simulink model "AUV_Model"  (R2019b)
settings: Solver=VariableStepAuto  StartTime=0.0  StopTime=300  FixedStep=0.5  RelTol=1e-3
InitFcn:
  | mdlWks = get_param(gcs,'ModelWorkspace');
  | a = getVariable(mdlWks,'a');
  | b = getVariable(mdlWks,'b');
  | c = getVariable(mdlWks,'c');
StopFcn:
  | figure(2)
  | plot3(Position_Data(1,1),Position_Data(1,2),Position_Data(1,3),'r*')
  | hold on
  | plot3(Position_Data(:,1),Position_Data(:,2),Position_Data(:,3));
  | plot3(Position_Data(end,1),Position_Data(end,2),Position_Data(end,3),'g*');
  | grid on
  | legend('Start Point','Trajectory','End Point')
model workspace (MAT data in the model file):
  a = 1
  b = 0
  c = 1
undefined symbols (not defined in the file): sigbuilder_block
libraries: simulink x6, sharedtransform x6, vrlib x6, dspfdesign x6, shared6dof x1, aerolibasang x1, aerolibnav x1
(part 2 of 3)

== system AUV_Model/ Translation Controller ==
  Actual Parameters : Inport
  Reference Parameters : Inport  Port=2
  Position Controller : Subsystem  VariantControl=a==0
  Velocity Controller : Subsystem  VariantControl=a==1
  Thrust Control : Outport  VectorParamsAs1DForOutWhenUnconnected=off

== system AUV_Model/Plant and Environment Model ==
  Thrust Control : Inport
  Combine Forces and Moments : Subsystem
  Dynamics solver : Subsystem
  Environmental Forces & Moments : Subsystem
  Propulsion Forces & Moments : Subsystem
  Outport : Outport  VectorParamsAs1DForOutWhenUnconnected=off
  wires:
  Thrust Control/1 -> Propulsion Forces & Moments/1(Thrust Control In)
  Propulsion Forces & Moments/1(Propulsion Parameters) -> Combine Forces and Moments/1(Propulsion Parameters)
  Environmental Forces & Moments/1(Environment Parameters) -> Combine Forces and Moments/2(Hydrodynamic Force)
  Combine Forces and Moments/1(Total Force) -> Dynamics solver/1(Total Force)
  Combine Forces and Moments/2(Total Moment) -> Dynamics solver/2(Total Moment)
  Dynamics solver/1(AUV Data) -> Outport/1
  Dynamics solver/2(Internal Parameters) -> Environmental Forces & Moments/1(AOA_SideSlip)

== system AUV_Model/Sensor data and State Estimation ==
  AUV_Parameters : Inport
  System With Noise : Subsystem  VariantControl=b==0
  System without Noise : Subsystem  VariantControl=b==1
  Filtered Parameters : Outport  VectorParamsAs1DForOutWhenUnconnected=off

== system AUV_Model/Switch Parameters ==
  Constant : Constant  Value=a
  Constant1 : Constant  Value=b
  Constant2 : Constant  Value=c
  Terminator1 : Terminator
  Terminator2 : Terminator
  Terminator3 : Terminator
  wires:
  Constant/1 -> Terminator1/1
  Constant1/1 -> Terminator2/1
  Constant2/1 -> Terminator3/1

== system AUV_Model/Translational Reference ==
  Bus Creator : BusCreator  Inputs=2
  Constant : Constant  Value=-10
  Constant1 : Constant  Value=0
  Mux : Mux  Inputs=3
  Mux1 : Mux  Inputs=3
  Signal Builder : Subsystem  Tag=STV Subsys  LoadFcn=sigbuilder_block('load');  StartFcn=sigbuilder_block('start');  StopFcn=sigbuilder_block('stop');  ClipboardFcn=sigbuilder_block('clipboard');  mask(Sigbuilder block){tuvar=[0:10]}
      mask help: Simulink:masks:SigbuilderBlock_MD
      mask init:
      | if ~strcmp(get_param(bdroot(gcbh),'SimulationStatus'),'stopped') tuvar = sigbuilder_block('maskInit'); end
      settings: CopyFcn=sigbuilder_block('copy');  DeleteFcn=sigbuilder_block('delete');  ModelCloseFcn=sigbuilder_block('modelClose');  PreSaveFcn=sigbuilder_block('preSave');  PauseFcn=sigbuilder_block('pause');  ContinueFcn=sigbuilder_block('continue');  NameChangeFcn=sigbuilder_block('namechange');  OpenFcn=sigbuilder_block('open',[49.5 -20.25 1204.5 394.5 ]);  CloseFcn=sigbuilder_block('close');
      mask Display: plot(0, 0, 100, 100,[2, 2, 32, 32, 2], [68, 8, 8, 68, 68],[32, 2], [38, 38], [32, 19, 2],[53, 60, 44], [32, 17, 17, 2],[16, 16, 31, 31]);txt = getActiveGroup(gcbh);text(2, 100, txt,'verticalAlignment', 'top');
  Step : Step  Time=30  Before=0.2  After=0  SampleTime=0
  Step1 : Step  Time=150  After=5  SampleTime=0
  Reference Parameters : Outport  VectorParamsAs1DForOutWhenUnconnected=off
  wires:
  Mux/1 -> Bus Creator/1  "Reference Position"
  Constant/1 -> Mux/1, Mux/2
  Step1/1 -> Mux/3
  Mux1/1 -> Bus Creator/2  "Reference Velocity"
  Bus Creator/1 -> Reference Parameters/1
  Signal Builder/1(Signal 2) -> Mux1/3
  Constant1/1 -> Mux1/2
  Step/1 -> Mux1/1

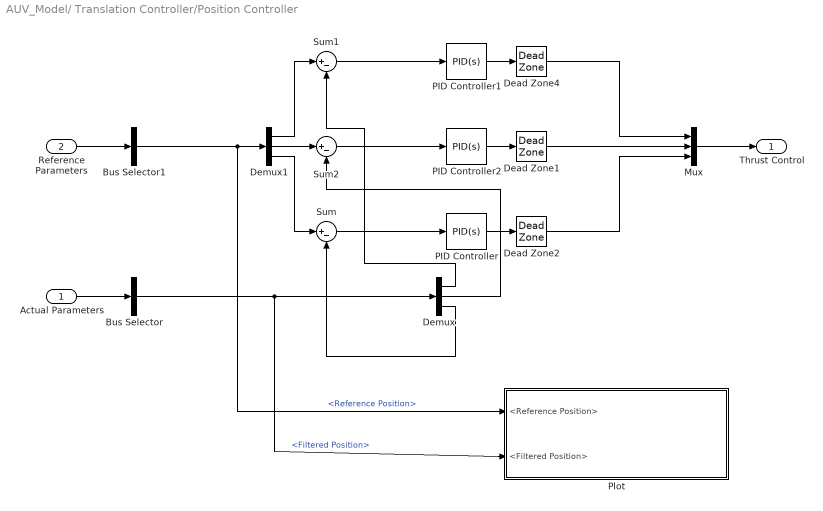
== system AUV_Model/ Translation Controller/Position Controller ==
  Actual Parameters : Inport
  Reference Parameters : Inport  Port=2
  Bus Selector : BusSelector  OutputSignals=Filtered Position
  Bus Selector1 : BusSelector  OutputSignals=Reference Position
  Dead Zone1 : DeadZone  LowerValue=-0.05  UpperValue=+0.05  SaturateOnIntegerOverflow=on
  Dead Zone2 : DeadZone  LowerValue=-0.05  UpperValue=+0.05  SaturateOnIntegerOverflow=on
  Dead Zone4 : DeadZone  LowerValue=-0.05  UpperValue=+0.05  SaturateOnIntegerOverflow=on
  Demux : Demux  Outputs=3
  Demux1 : Demux  Outputs=3
  Mux : Mux  Inputs=3
  PID Controller : simulink/Continuous/PID Controller  Controller=PID  Form=Parallel  TimeDomain=Continuous-time  SampleTime=-1  IntegratorMethod=Forward Euler  FilterMethod=Forward Euler  ControllerParametersSource=internal  P=-0.0440831016133051  I=-0.00046335965727533  D=-0.931852208113014  UseFilter=on  N=205.904485551143  TunerSelectOption=Transfer Function Based (PID Tuner App)  InitialConditionSource=internal  InitialConditionForIntegrator=0  InitialConditionForFilter=0  DifferentiatorICPrevScaledInput=0  ExternalReset=none  TrackingMode=off  Kt=1  LimitOutput=off  UpperSaturationLimit=inf  LowerSaturationLimit=-inf  LinearizeAsGain=on  AntiWindupMode=none  Kb=1  POutMin=[]  POutMax=[]  IOutMin=[]  IOutMax=[]  DOutMin=[]  DOutMax=[]  NOutMin=[]  NOutMax=[]  SumOutMin=[]  SumOutMax=[]  SaturationOutMin=[]  SaturationOutMax=[]  PParamMin=[]  PParamMax=[]  IParamMin=[]  IParamMax=[]  DParamMin=[]  DParamMax=[]  NParamMin=[]  NParamMax=[]  KbParamMin=[]  KbParamMax=[]  KtParamMin=[]  KtParamMax=[]  KbOutMin=[]  KbOutMax=[]  KtOutMin=[]  KtOutMax=[]  IntegratorOutMin=[]  IntegratorOutMax=[]  FilterOutMin=[]  FilterOutMax=[]  SumI1OutMin=[]  SumI1OutMax=[]  SumI2OutMin=[]  SumI2OutMax=[]  SumI3OutMin=[]  SumI3OutMax=[]  SumI4OutMin=[]  SumI4OutMax=[]  SumDOutMin=[]  SumDOutMax=[]  DifferentiatorOutMin=[]  DifferentiatorOutMax=[]  FilterDiffOutCoefMin=[]  FilterDiffOutCoefMax=[]  ReciprocalOutMin=[]  ReciprocalOutMax=[]  SumDenOutMin=[]  SumDenOutMax=[]  SumNumOutMin=[]  SumNumOutMax=[]  DivideOutMin=[]  DivideOutMax=[]  IntegratorContinuousStateAttributes=''  IntegratorStateMustResolveToSignalObject=off  IntegratorRTWStateStorageClass=Auto  FilterContinuousStateAttributes=''  FilterStateMustResolveToSignalObject=off  FilterRTWStateStorageClass=Auto  ParallelPVariant=InternalParameters  IdealPVariant=Disabled  IVariant=InternalParameters  DVariant=InternalParameters  IntegratorVariant=Continuous  SatVariant=Disabled  AWVariant=Passthrough  PCopyVariant=Disabled  TRVariant=Disabled  FdbkBlocksVariant=Forward  IdealPFdbkVariant=Disabled  SatFdbkVariant=Disabled  DerivativeFilterVariant=ContFilter  NVariant=InternalParameters  NCopyVariant=Disabled  FilterICVariant=InternalICsFilter  IntegratorICVariant=InternalICs  ExternalResetVariant=Disabled  TRSumVariant=Passthrough  SumFdbkVariant=Disabled  SumVariant=Sum_PID
  PID Controller1 : simulink/Continuous/PID Controller  Controller=PID  Form=Parallel  TimeDomain=Continuous-time  SampleTime=-1  IntegratorMethod=Forward Euler  FilterMethod=Forward Euler  ControllerParametersSource=internal  P=0.0352909553215239  I=0.000468513300704798  D=0.59064410837381  UseFilter=on  N=260.062804539004  TunerSelectOption=Transfer Function Based (PID Tuner App)  InitialConditionSource=internal  InitialConditionForIntegrator=0  InitialConditionForFilter=0  DifferentiatorICPrevScaledInput=0  ExternalReset=none  TrackingMode=off  Kt=1  LimitOutput=off  UpperSaturationLimit=inf  LowerSaturationLimit=-inf  LinearizeAsGain=on  AntiWindupMode=none  Kb=1  POutMin=[]  POutMax=[]  IOutMin=[]  IOutMax=[]  DOutMin=[]  DOutMax=[]  NOutMin=[]  NOutMax=[]  SumOutMin=[]  SumOutMax=[]  SaturationOutMin=[]  SaturationOutMax=[]  PParamMin=[]  PParamMax=[]  IParamMin=[]  IParamMax=[]  DParamMin=[]  DParamMax=[]  NParamMin=[]  NParamMax=[]  KbParamMin=[]  KbParamMax=[]  KtParamMin=[]  KtParamMax=[]  KbOutMin=[]  KbOutMax=[]  KtOutMin=[]  KtOutMax=[]  IntegratorOutMin=[]  IntegratorOutMax=[]  FilterOutMin=[]  FilterOutMax=[]  SumI1OutMin=[]  SumI1OutMax=[]  SumI2OutMin=[]  SumI2OutMax=[]  SumI3OutMin=[]  SumI3OutMax=[]  SumI4OutMin=[]  SumI4OutMax=[]  SumDOutMin=[]  SumDOutMax=[]  DifferentiatorOutMin=[]  DifferentiatorOutMax=[]  FilterDiffOutCoefMin=[]  FilterDiffOutCoefMax=[]  ReciprocalOutMin=[]  ReciprocalOutMax=[]  SumDenOutMin=[]  SumDenOutMax=[]  SumNumOutMin=[]  SumNumOutMax=[]  DivideOutMin=[]  DivideOutMax=[]  IntegratorContinuousStateAttributes=''  IntegratorStateMustResolveToSignalObject=off  IntegratorRTWStateStorageClass=Auto  FilterContinuousStateAttributes=''  FilterStateMustResolveToSignalObject=off  FilterRTWStateStorageClass=Auto  ParallelPVariant=InternalParameters  IdealPVariant=Disabled  IVariant=InternalParameters  DVariant=InternalParameters  IntegratorVariant=Continuous  SatVariant=Disabled  AWVariant=Passthrough  PCopyVariant=Disabled  TRVariant=Disabled  FdbkBlocksVariant=Forward  IdealPFdbkVariant=Disabled  SatFdbkVariant=Disabled  DerivativeFilterVariant=ContFilter  NVariant=InternalParameters  NCopyVariant=Disabled  FilterICVariant=InternalICsFilter  IntegratorICVariant=InternalICs  ExternalResetVariant=Disabled  TRSumVariant=Passthrough  SumFdbkVariant=Disabled  SumVariant=Sum_PID
  PID Controller2 : simulink/Continuous/PID Controller  Controller=PID  Form=Parallel  TimeDomain=Continuous-time  SampleTime=-1  IntegratorMethod=Forward Euler  FilterMethod=Forward Euler  ControllerParametersSource=internal  P=0.172975950646219  I=0.00387308418128247  D=1.71646711354372  UseFilter=on  N=438.622536688858  TunerSelectOption=Transfer Function Based (PID Tuner App)  InitialConditionSource=internal  InitialConditionForIntegrator=0  InitialConditionForFilter=0  DifferentiatorICPrevScaledInput=0  ExternalReset=none  TrackingMode=off  Kt=1  LimitOutput=off  UpperSaturationLimit=inf  LowerSaturationLimit=-inf  LinearizeAsGain=on  AntiWindupMode=none  Kb=1  POutMin=[]  POutMax=[]  IOutMin=[]  IOutMax=[]  DOutMin=[]  DOutMax=[]  NOutMin=[]  NOutMax=[]  SumOutMin=[]  SumOutMax=[]  SaturationOutMin=[]  SaturationOutMax=[]  PParamMin=[]  PParamMax=[]  IParamMin=[]  IParamMax=[]  DParamMin=[]  DParamMax=[]  NParamMin=[]  NParamMax=[]  KbParamMin=[]  KbParamMax=[]  KtParamMin=[]  KtParamMax=[]  KbOutMin=[]  KbOutMax=[]  KtOutMin=[]  KtOutMax=[]  IntegratorOutMin=[]  IntegratorOutMax=[]  FilterOutMin=[]  FilterOutMax=[]  SumI1OutMin=[]  SumI1OutMax=[]  SumI2OutMin=[]  SumI2OutMax=[]  SumI3OutMin=[]  SumI3OutMax=[]  SumI4OutMin=[]  SumI4OutMax=[]  SumDOutMin=[]  SumDOutMax=[]  DifferentiatorOutMin=[]  DifferentiatorOutMax=[]  FilterDiffOutCoefMin=[]  FilterDiffOutCoefMax=[]  ReciprocalOutMin=[]  ReciprocalOutMax=[]  SumDenOutMin=[]  SumDenOutMax=[]  SumNumOutMin=[]  SumNumOutMax=[]  DivideOutMin=[]  DivideOutMax=[]  IntegratorContinuousStateAttributes=''  IntegratorStateMustResolveToSignalObject=off  IntegratorRTWStateStorageClass=Auto  FilterContinuousStateAttributes=''  FilterStateMustResolveToSignalObject=off  FilterRTWStateStorageClass=Auto  ParallelPVariant=InternalParameters  IdealPVariant=Disabled  IVariant=InternalParameters  DVariant=InternalParameters  IntegratorVariant=Continuous  SatVariant=Disabled  AWVariant=Passthrough  PCopyVariant=Disabled  TRVariant=Disabled  FdbkBlocksVariant=Forward  IdealPFdbkVariant=Disabled  SatFdbkVariant=Disabled  DerivativeFilterVariant=ContFilter  NVariant=InternalParameters  NCopyVariant=Disabled  FilterICVariant=InternalICsFilter  IntegratorICVariant=InternalICs  ExternalResetVariant=Disabled  TRSumVariant=Passthrough  SumFdbkVariant=Disabled  SumVariant=Sum_PID
  Plot : Subsystem
  Sum : Sum  Inputs=|+-
  Sum1 : Sum  Inputs=|+-
  Sum2 : Sum  Inputs=|+-
  Thrust Control : Outport  VectorParamsAs1DForOutWhenUnconnected=off
  wires:
  Demux1/1 -> Sum1/1
  Demux1/3 -> Sum/1
  Demux1/2 -> Sum2/1
  PID Controller1/1 -> Dead Zone4/1
  Demux/3 -> Sum/2
  PID Controller2/1 -> Dead Zone1/1
  Demux/2 -> Sum2/2
  Sum2/1 -> PID Controller2/1
  Demux/1 -> Sum1/2
  Sum/1 -> PID Controller/1
  PID Controller/1 -> Dead Zone2/1
  Sum1/1 -> PID Controller1/1
  Mux/1 -> Thrust Control/1
  Dead Zone4/1 -> Mux/1
  Dead Zone1/1 -> Mux/2
  Dead Zone2/1 -> Mux/3
  Actual Parameters/1 -> Bus Selector/1
  Bus Selector/1 -> Plot/2(<Filtered Position>), Demux/1  "<Filtered Position>"
  Reference Parameters/1 -> Bus Selector1/1
  Bus Selector1/1 -> Plot/1(<Reference Position>), Demux1/1  "<Reference Position>"

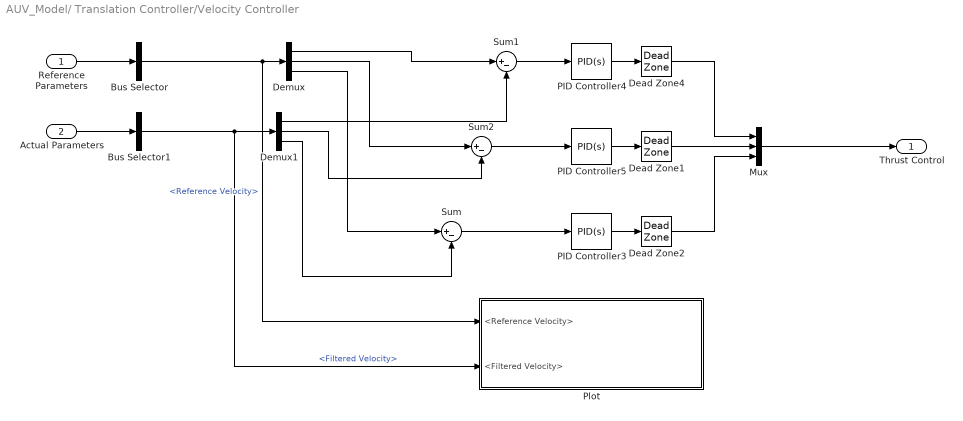
== system AUV_Model/ Translation Controller/Velocity Controller ==
  Reference Parameters : Inport
  Actual Parameters : Inport  Port=2
  Bus Selector : BusSelector  OutputSignals=Reference Velocity
  Bus Selector1 : BusSelector  OutputSignals=Filtered Velocity
  Dead Zone1 : DeadZone  LowerValue=-0.05  UpperValue=+0.05  SaturateOnIntegerOverflow=on
  Dead Zone2 : DeadZone  LowerValue=-0.05  UpperValue=+0.05  SaturateOnIntegerOverflow=on
  Dead Zone4 : DeadZone  LowerValue=-0.05  UpperValue=+0.05  SaturateOnIntegerOverflow=on
  Demux : Demux  Outputs=3
  Demux1 : Demux  Outputs=3
  Mux : Mux  Inputs=3
  PID Controller3 : simulink/Continuous/PID Controller  Controller=PID  Form=Parallel  TimeDomain=Continuous-time  SampleTime=-1  IntegratorMethod=Forward Euler  FilterMethod=Forward Euler  ControllerParametersSource=internal  P=-0.61964554396314  I=-0.140214385843897  D=0.00440045709674139  UseFilter=on  N=140.813904178727  TunerSelectOption=Transfer Function Based (PID Tuner App)  InitialConditionSource=internal  InitialConditionForIntegrator=0  InitialConditionForFilter=0  DifferentiatorICPrevScaledInput=0  ExternalReset=none  TrackingMode=off  Kt=1  LimitOutput=off  UpperSaturationLimit=inf  LowerSaturationLimit=-inf  LinearizeAsGain=on  AntiWindupMode=none  Kb=1  POutMin=[]  POutMax=[]  IOutMin=[]  IOutMax=[]  DOutMin=[]  DOutMax=[]  NOutMin=[]  NOutMax=[]  SumOutMin=[]  SumOutMax=[]  SaturationOutMin=[]  SaturationOutMax=[]  PParamMin=[]  PParamMax=[]  IParamMin=[]  IParamMax=[]  DParamMin=[]  DParamMax=[]  NParamMin=[]  NParamMax=[]  KbParamMin=[]  KbParamMax=[]  KtParamMin=[]  KtParamMax=[]  KbOutMin=[]  KbOutMax=[]  KtOutMin=[]  KtOutMax=[]  IntegratorOutMin=[]  IntegratorOutMax=[]  FilterOutMin=[]  FilterOutMax=[]  SumI1OutMin=[]  SumI1OutMax=[]  SumI2OutMin=[]  SumI2OutMax=[]  SumI3OutMin=[]  SumI3OutMax=[]  SumI4OutMin=[]  SumI4OutMax=[]  SumDOutMin=[]  SumDOutMax=[]  DifferentiatorOutMin=[]  DifferentiatorOutMax=[]  FilterDiffOutCoefMin=[]  FilterDiffOutCoefMax=[]  ReciprocalOutMin=[]  ReciprocalOutMax=[]  SumDenOutMin=[]  SumDenOutMax=[]  SumNumOutMin=[]  SumNumOutMax=[]  DivideOutMin=[]  DivideOutMax=[]  IntegratorContinuousStateAttributes=''  IntegratorStateMustResolveToSignalObject=off  IntegratorRTWStateStorageClass=Auto  FilterContinuousStateAttributes=''  FilterStateMustResolveToSignalObject=off  FilterRTWStateStorageClass=Auto  ParallelPVariant=InternalParameters  IdealPVariant=Disabled  IVariant=InternalParameters  DVariant=InternalParameters  IntegratorVariant=Continuous  SatVariant=Disabled  AWVariant=Passthrough  PCopyVariant=Disabled  TRVariant=Disabled  FdbkBlocksVariant=Forward  IdealPFdbkVariant=Disabled  SatFdbkVariant=Disabled  DerivativeFilterVariant=ContFilter  NVariant=InternalParameters  NCopyVariant=Disabled  FilterICVariant=InternalICsFilter  IntegratorICVariant=InternalICs  ExternalResetVariant=Disabled  TRSumVariant=Passthrough  SumFdbkVariant=Disabled  SumVariant=Sum_PID
  PID Controller4 : simulink/Continuous/PID Controller  Controller=PID  Form=Parallel  TimeDomain=Continuous-time  SampleTime=-1  IntegratorMethod=Forward Euler  FilterMethod=Forward Euler  ControllerParametersSource=internal  P=0.262050505979025  I=0.0518732197045156  D=-0.0235509594288088  UseFilter=on  N=11.1269567072699  TunerSelectOption=Transfer Function Based (PID Tuner App)  InitialConditionSource=internal  InitialConditionForIntegrator=0  InitialConditionForFilter=0  DifferentiatorICPrevScaledInput=0  ExternalReset=none  TrackingMode=off  Kt=1  LimitOutput=off  UpperSaturationLimit=inf  LowerSaturationLimit=-inf  LinearizeAsGain=on  AntiWindupMode=none  Kb=1  POutMin=[]  POutMax=[]  IOutMin=[]  IOutMax=[]  DOutMin=[]  DOutMax=[]  NOutMin=[]  NOutMax=[]  SumOutMin=[]  SumOutMax=[]  SaturationOutMin=[]  SaturationOutMax=[]  PParamMin=[]  PParamMax=[]  IParamMin=[]  IParamMax=[]  DParamMin=[]  DParamMax=[]  NParamMin=[]  NParamMax=[]  KbParamMin=[]  KbParamMax=[]  KtParamMin=[]  KtParamMax=[]  KbOutMin=[]  KbOutMax=[]  KtOutMin=[]  KtOutMax=[]  IntegratorOutMin=[]  IntegratorOutMax=[]  FilterOutMin=[]  FilterOutMax=[]  SumI1OutMin=[]  SumI1OutMax=[]  SumI2OutMin=[]  SumI2OutMax=[]  SumI3OutMin=[]  SumI3OutMax=[]  SumI4OutMin=[]  SumI4OutMax=[]  SumDOutMin=[]  SumDOutMax=[]  DifferentiatorOutMin=[]  DifferentiatorOutMax=[]  FilterDiffOutCoefMin=[]  FilterDiffOutCoefMax=[]  ReciprocalOutMin=[]  ReciprocalOutMax=[]  SumDenOutMin=[]  SumDenOutMax=[]  SumNumOutMin=[]  SumNumOutMax=[]  DivideOutMin=[]  DivideOutMax=[]  IntegratorContinuousStateAttributes=''  IntegratorStateMustResolveToSignalObject=off  IntegratorRTWStateStorageClass=Auto  FilterContinuousStateAttributes=''  FilterStateMustResolveToSignalObject=off  FilterRTWStateStorageClass=Auto  ParallelPVariant=InternalParameters  IdealPVariant=Disabled  IVariant=InternalParameters  DVariant=InternalParameters  IntegratorVariant=Continuous  SatVariant=Disabled  AWVariant=Passthrough  PCopyVariant=Disabled  TRVariant=Disabled  FdbkBlocksVariant=Forward  IdealPFdbkVariant=Disabled  SatFdbkVariant=Disabled  DerivativeFilterVariant=ContFilter  NVariant=InternalParameters  NCopyVariant=Disabled  FilterICVariant=InternalICsFilter  IntegratorICVariant=InternalICs  ExternalResetVariant=Disabled  TRSumVariant=Passthrough  SumFdbkVariant=Disabled  SumVariant=Sum_PID
  PID Controller5 : simulink/Continuous/PID Controller  Controller=PID  Form=Parallel  TimeDomain=Continuous-time  SampleTime=-1  IntegratorMethod=Forward Euler  FilterMethod=Forward Euler  ControllerParametersSource=internal  P=1.14371295451496  I=0.548529610159355  D=-0.00383210771245667  UseFilter=on  N=298.455325458939  TunerSelectOption=Transfer Function Based (PID Tuner App)  InitialConditionSource=internal  InitialConditionForIntegrator=0  InitialConditionForFilter=0  DifferentiatorICPrevScaledInput=0  ExternalReset=none  TrackingMode=off  Kt=1  LimitOutput=off  UpperSaturationLimit=inf  LowerSaturationLimit=-inf  LinearizeAsGain=on  AntiWindupMode=none  Kb=1  POutMin=[]  POutMax=[]  IOutMin=[]  IOutMax=[]  DOutMin=[]  DOutMax=[]  NOutMin=[]  NOutMax=[]  SumOutMin=[]  SumOutMax=[]  SaturationOutMin=[]  SaturationOutMax=[]  PParamMin=[]  PParamMax=[]  IParamMin=[]  IParamMax=[]  DParamMin=[]  DParamMax=[]  NParamMin=[]  NParamMax=[]  KbParamMin=[]  KbParamMax=[]  KtParamMin=[]  KtParamMax=[]  KbOutMin=[]  KbOutMax=[]  KtOutMin=[]  KtOutMax=[]  IntegratorOutMin=[]  IntegratorOutMax=[]  FilterOutMin=[]  FilterOutMax=[]  SumI1OutMin=[]  SumI1OutMax=[]  SumI2OutMin=[]  SumI2OutMax=[]  SumI3OutMin=[]  SumI3OutMax=[]  SumI4OutMin=[]  SumI4OutMax=[]  SumDOutMin=[]  SumDOutMax=[]  DifferentiatorOutMin=[]  DifferentiatorOutMax=[]  FilterDiffOutCoefMin=[]  FilterDiffOutCoefMax=[]  ReciprocalOutMin=[]  ReciprocalOutMax=[]  SumDenOutMin=[]  SumDenOutMax=[]  SumNumOutMin=[]  SumNumOutMax=[]  DivideOutMin=[]  DivideOutMax=[]  IntegratorContinuousStateAttributes=''  IntegratorStateMustResolveToSignalObject=off  IntegratorRTWStateStorageClass=Auto  FilterContinuousStateAttributes=''  FilterStateMustResolveToSignalObject=off  FilterRTWStateStorageClass=Auto  ParallelPVariant=InternalParameters  IdealPVariant=Disabled  IVariant=InternalParameters  DVariant=InternalParameters  IntegratorVariant=Continuous  SatVariant=Disabled  AWVariant=Passthrough  PCopyVariant=Disabled  TRVariant=Disabled  FdbkBlocksVariant=Forward  IdealPFdbkVariant=Disabled  SatFdbkVariant=Disabled  DerivativeFilterVariant=ContFilter  NVariant=InternalParameters  NCopyVariant=Disabled  FilterICVariant=InternalICsFilter  IntegratorICVariant=InternalICs  ExternalResetVariant=Disabled  TRSumVariant=Passthrough  SumFdbkVariant=Disabled  SumVariant=Sum_PID
  Plot : Subsystem
  Sum : Sum  Inputs=|+-
  Sum1 : Sum  Inputs=|+-
  Sum2 : Sum  Inputs=|+-
  Thrust Control : Outport  VectorParamsAs1DForOutWhenUnconnected=off
  wires:
  Demux1/3 -> Sum/2
  PID Controller3/1 -> Dead Zone2/1
  Demux/3 -> Sum/1
  PID Controller4/1 -> Dead Zone4/1
  PID Controller5/1 -> Dead Zone1/1
  Demux/2 -> Sum2/1
  Dead Zone2/1 -> Mux/3
  Dead Zone1/1 -> Mux/2
  Demux/1 -> Sum1/1
  Demux1/1 -> Sum1/2
  Demux1/2 -> Sum2/2
  Dead Zone4/1 -> Mux/1
  Mux/1 -> Thrust Control/1
  Sum1/1 -> PID Controller4/1
  Sum2/1 -> PID Controller5/1
  Sum/1 -> PID Controller3/1
  Bus Selector/1 -> Plot/1(<Reference Velocity>), Demux/1  "<Reference Velocity>"
  Reference Parameters/1 -> Bus Selector/1
  Bus Selector1/1 -> Plot/2(<Filtered Velocity>), Demux1/1  "<Filtered Velocity>"
  Actual Parameters/1 -> Bus Selector1/1

== system AUV_Model/Plant and Environment Model/Combine Forces and Moments ==
  Propulsion Parameters : Inport
  Hydrodynamic Force : Inport  Port=2
  Bus Selector : BusSelector  OutputSignals=PropForce,PropMoment
  Bus Selector1 : BusSelector  OutputSignals=LDForce,HSForce,HS Moment
  Saturation : Saturate  UpperLimit=600  LowerLimit=-600
  Saturation1 : Saturate  UpperLimit=600  LowerLimit=-600
  Sum : Sum  Inputs=+++
  Sum1 : Sum  Inputs=|++
  Total Force : Outport  VectorParamsAs1DForOutWhenUnconnected=off
  Total Moment : Outport  Port=2  VectorParamsAs1DForOutWhenUnconnected=off
  wires:
  Bus Selector1/3 -> Sum1/2  "<HS Moment>"
  Bus Selector/2 -> Sum1/1  "<PropMoment>"
  Sum/1 -> Saturation/1
  Sum1/1 -> Total Moment/1
  Saturation1/1 -> Sum/2
  Saturation/1 -> Total Force/1
  Propulsion Parameters/1 -> Bus Selector/1
  Hydrodynamic Force/1 -> Bus Selector1/1
  Bus Selector/1 -> Sum/1  "<PropForce>"
  Bus Selector1/1 -> Saturation1/1  "<LDForce>"
  Bus Selector1/2 -> Sum/3  "<HSForce>"

== system AUV_Model/Plant and Environment Model/Dynamics solver ==
  Total Force : Inport
  Total Moment : Inport  Port=2
  6DOF (Euler Angles) : shared6dof/6DOF (Euler Angles)  units=Metric (MKS)  mtype=Fixed  rep=Euler Angles  xme_0=[0.01 .01 .01]  Vm_0=[0.01 0.01 0.001]  eul_0=[0.001 0.001 0.001]  pm_0=[0.001 0.001 0.001]  mass_0=10  mass_e=0.5  mass_f=2.0  inertia=10*eye(3)  inertia_e=eye(3)  inertia_f=2*eye(3)  k_quat=1.0  vre_flag=on  abi_flag=on  aMode=0  xme_statename=''  Vm_statename=''  eul_statename=''  quat_statename=''  pm_statename=''  mass_statename=''
      settings: SourceProductBaseCode=AE
  Bus Creator : BusCreator  Inputs=4
  Bus Creator1 : BusCreator  Inputs=3
  Post-Processing : Subsystem
  Terminator : Terminator
  Terminator1 : Terminator
  AUV Data : Outport  VectorParamsAs1DForOutWhenUnconnected=off
  Internal Parameters : Outport  Port=2  VectorParamsAs1DForOutWhenUnconnected=off
  wires:
  6DOF (Euler Angles)/6 -> Post-Processing/4(Body angular rates)  "Body_rates"
  Post-Processing/3("AOA, Side slip") -> Bus Creator1/2  "AOA_SS"
  6DOF (Euler Angles)/8 -> Post-Processing/6(Body Acceleration)  "Body_acc"
  Post-Processing/2(" Position") -> Bus Creator/2  "Position"
  6DOF (Euler Angles)/7 -> Post-Processing/5(Body angular accelerations)  "Body_ang_acc"
  6DOF (Euler Angles)/2 -> Post-Processing/2(Position (Reference Frame))  "Pos_Ref"
  6DOF (Euler Angles)/3 -> Post-Processing/3(Orientation angles)  "Body_Angles"
  Post-Processing/1(Velocity) -> Bus Creator/1  "Velocity"
  6DOF (Euler Angles)/1 -> Post-Processing/1(Velocity (Reference Frame))  "Velocity_Ref"
  6DOF (Euler Angles)/5 -> Bus Creator1/3, Post-Processing/7(Body velocity)  "Velocity_body"
  Post-Processing/4(Orientation Angles) -> Bus Creator1/1, Bus Creator/3  "Orientation Angles"
  Post-Processing/5(IMU Data) -> Bus Creator/4  "IMU Data"
  Total Force/1 -> 6DOF (Euler Angles)/1
  Total Moment/1 -> 6DOF (Euler Angles)/2
  Bus Creator/1 -> AUV Data/1
  Bus Creator1/1 -> Internal Parameters/1
  6DOF (Euler Angles)/4 -> Terminator/1
  6DOF (Euler Angles)/9 -> Terminator1/1

== system AUV_Model/Plant and Environment Model/Environmental Forces & Moments ==
  AOA_SideSlip : Inport
  Bus Creator : BusCreator  Inputs=3
  Bus Selector : BusSelector  OutputSignals=Velocity_body,AOA_SS,Orientation Angles
  Hydrodynamic Forces : Subsystem  Variant=on
  Hydrostatic Forces : Subsystem
  Environment Parameters : Outport  VectorParamsAs1DForOutWhenUnconnected=off
  wires:
  Hydrodynamic Forces/1("Force due to Lift, Drag") -> Bus Creator/1  "LDForce"
  Hydrostatic Forces/1(Hydrostatic Force) -> Bus Creator/2  "HSForce"
  Hydrostatic Forces/2(Hydrostatic Moment) -> Bus Creator/3  "HS Moment"
  Bus Creator/1 -> Environment Parameters/1
  AOA_SideSlip/1 -> Bus Selector/1
  Bus Selector/1 -> Hydrodynamic Forces/1("Submarine Velocity (Body Axis) ")  "<Velocity_body>"
  Bus Selector/2 -> Hydrodynamic Forces/2("AOA, Side Slip")  "<AOA_SS>"
  Bus Selector/3 -> Hydrostatic Forces/1(In1)  "<Orientation Angles>"

== system AUV_Model/Plant and Environment Model/Propulsion Forces & Moments ==
  Thrust Control In : Inport
  Bus Creator : BusCreator  Inputs=2
  Force and moments due to Thrust : Subsystem
  Input commands to Thrust : Subsystem
  Propulsion Parameters : Outport  VectorParamsAs1DForOutWhenUnconnected=off
  wires:
  Input commands to Thrust/1(Thrust values) -> Force and moments due to Thrust/1(Thrust Inputs)
  Thrust Control In/1 -> Input commands to Thrust/1(Thrust Control Inputs)
  Force and moments due to Thrust/1(Propulsion Force) -> Bus Creator/1  "PropForce"
  Force and moments due to Thrust/2(Propulsion Moment) -> Bus Creator/2  "PropMoment"
  Bus Creator/1 -> Propulsion Parameters/1

== system AUV_Model/Sensor data and State Estimation/System With Noise ==
  AUV_Parameters : Inport
  " Sensor (IMU)" : Subsystem
  Internal filter : Subsystem
  Filtered Parameters : Outport  VectorParamsAs1DForOutWhenUnconnected=off
  wires:
  AUV_Parameters/1 -> " Sensor (IMU)"/1(IMU Inputs)
  Internal filter/1(Filtered Parameters) -> Filtered Parameters/1
  " Sensor (IMU)"/1(IMU Measurements) -> Internal filter/1(Accel)

== system AUV_Model/Sensor data and State Estimation/System without Noise ==
  AUV_Parameters : Inport
  Bus Creator : BusCreator  Inputs=2
  Bus Selector : BusSelector  OutputSignals=Position,Velocity
  Gain : Gain
  Gain1 : Gain
  Filtered Parameters : Outport  VectorParamsAs1DForOutWhenUnconnected=off
  wires:
  Bus Creator/1 -> Filtered Parameters/1
  Bus Selector/2 -> Gain1/1  "<Velocity>"
  Bus Selector/1 -> Gain/1  "<Position>"
  Gain1/1 -> Bus Creator/2  "Filtered Velocity"
  Gain/1 -> Bus Creator/1  "Filtered Position"
  AUV_Parameters/1 -> Bus Selector/1

== system AUV_Model/Translational Reference/Signal Builder ==
  Demux : Demux  Tag=STV Demux  Outputs=1
  FromWs : FromWorkspace  Tag=STV FromWs  VariableName=tuvar  SampleTime=0
      SigBuilderData=|
      | common.afterFinalStr = 'Extrapolate'
      | common.sampleTime = 0
      | dataSet.timeRange = [0 300]
      | dataSet.name = 'Group 1'
      | sbobj.Groups.Name = 'Group 1'
      | sbobj.Groups.Signals.Name = 'Signal 2'
      | sbobj.Groups.Signals.XData = [0 150 150 180 180 300]
      | sbobj.Groups.Signals.YData = [0 0 0.2 0.2 0 0]
      | sbobj.Groups.TimeRange = [0 300]
  Signal 2 : Outport  Tag=STV Outport  VectorParamsAs1DForOutWhenUnconnected=off
  wires:
  FromWs/1 -> Demux/1
  Demux/1 -> Signal 2/1

== system AUV_Model/ Translation Controller/Position Controller/Plot ==
  <Reference Position> : Inport
  <Filtered Position> : Inport  Port=2
  Demux2 : Demux  Outputs=3
  Demux3 : Demux  Outputs=3
  Mux1 : Mux  Inputs=2
  Mux2 : Mux  Inputs=2
  Mux3 : Mux  Inputs=2
  Scope : Scope  NumInputPorts=3
  wires:
  Mux3/1 -> Scope/3
  Demux3/1 -> Mux1/2
  Demux3/2 -> Mux2/2
  Demux2/3 -> Mux3/1
  Mux2/1 -> Scope/2
  Mux1/1 -> Scope/1
  Demux2/2 -> Mux2/1
  Demux2/1 -> Mux1/1
  Demux3/3 -> Mux3/2
  <Reference Position>/1 -> Demux2/1
  <Filtered Position>/1 -> Demux3/1

== system AUV_Model/ Translation Controller/Velocity Controller/Plot ==
  <Reference Velocity> : Inport
  <Filtered Velocity> : Inport  Port=2
  Demux2 : Demux  Outputs=3
  Demux3 : Demux  Outputs=3
  Mux1 : Mux  Inputs=2
  Mux2 : Mux  Inputs=2
  Mux3 : Mux  Inputs=2
  Scope : Scope  NumInputPorts=3
  wires:
  Mux3/1 -> Scope/3
  Demux3/1 -> Mux1/2
  Demux3/2 -> Mux2/2
  Demux2/3 -> Mux3/1
  Mux2/1 -> Scope/2
  Mux1/1 -> Scope/1
  Demux2/2 -> Mux2/1
  Demux2/1 -> Mux1/1
  Demux3/3 -> Mux3/2
  <Reference Velocity>/1 -> Demux2/1
  <Filtered Velocity>/1 -> Demux3/1

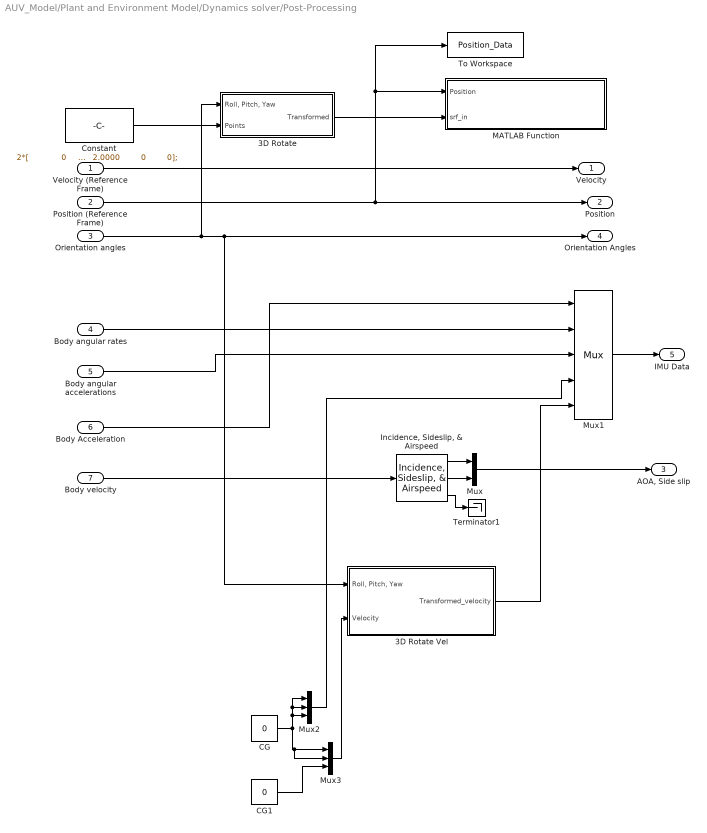
== system AUV_Model/Plant and Environment Model/Dynamics solver/Post-Processing ==
  Velocity (Reference Frame) : Inport
  Position (Reference Frame) : Inport  Port=2
  Orientation angles : Inport  Port=3
  Body angular rates : Inport  Port=4
  Body angular accelerations : Inport  Port=5
  Body Acceleration : Inport  Port=6
  Body velocity : Inport  Port=7
  "3D Rotate " : Subsystem
  3D Rotate Vel : Subsystem
  CG : Constant  Value=0
  CG1 : Constant  Value=0
  Constant : Constant  Value=|
      | 2*[              0         0         0
      |     2.0000         0         0
      |     2.0000    0.4000         0
      |          0    0.4000         0
      |          0         0         0
      |          0         0    0.4000
      |     2.0000         0    0.4000
      |     2.0000    0.4000    0.4000
      |          0    0.4000    0.4000
      |          0         0    0.4000
      |          0    0.4000    0.4000
      |          0    0.4000         0
      |     2.0000    0.4000         0
      |     2.0000    0.4000    0.4000
      |     2.0000         0    0.4000
      |     2.0000         0         0];
  "Incidence, Sideslip, & Airspeed" : aerolibasang/Incidence, Sideslip, & Airspeed
      settings: SourceProductName=Aerospace Blockset
  MATLAB Function : MATLAB Function  TreatAsAtomicUnit=on  SystemSampleTime=0.05
  Mux : Mux  Inputs=2
  Mux1 : Mux  Inputs=5
  Mux2 : Mux  Inputs=3
  Mux3 : Mux  Inputs=3
  Terminator1 : Terminator
  To Workspace : ToWorkspace  VariableName=Position_Data  SampleTime=-1
  Velocity : Outport  VectorParamsAs1DForOutWhenUnconnected=off
  " Position" : Outport  Port=2  VectorParamsAs1DForOutWhenUnconnected=off
  "AOA, Side slip" : Outport  Port=3  VectorParamsAs1DForOutWhenUnconnected=off
  Orientation Angles : Outport  Port=4  VectorParamsAs1DForOutWhenUnconnected=off
  IMU Data : Outport  Port=5  VectorParamsAs1DForOutWhenUnconnected=off
  wires:
  Body angular accelerations/1 -> Mux1/3
  "Incidence, Sideslip, & Airspeed"/2 -> Mux/2
  Body velocity/1 -> "Incidence, Sideslip, & Airspeed"/1
  "Incidence, Sideslip, & Airspeed"/1 -> Mux/1
  Body angular rates/1 -> Mux1/2
  CG/1 -> Mux2/3, Mux2/2, Mux2/1, Mux3/2, Mux3/1
  3D Rotate Vel/1("Transformed_velocity ") -> Mux1/5
  Mux2/1 -> Mux1/4
  Position (Reference Frame)/1 -> To Workspace/1, MATLAB Function/1(Position), " Position"/1
  Mux/1 -> "AOA, Side slip"/1
  CG1/1 -> Mux3/3
  Mux3/1 -> 3D Rotate Vel/2(Velocity)
  Body Acceleration/1 -> Mux1/1
  Velocity (Reference Frame)/1 -> Velocity/1
  Orientation angles/1 -> 3D Rotate Vel/1("Roll, Pitch, Yaw"), Orientation Angles/1, "3D Rotate "/1("Roll, Pitch, Yaw")
  Mux1/1 -> IMU Data/1
  Constant/1 -> "3D Rotate "/2(Points)
  "3D Rotate "/1("Transformed ") -> MATLAB Function/2(srf_in)
  "Incidence, Sideslip, & Airspeed"/3 -> Terminator1/1

== system AUV_Model/Plant and Environment Model/Environmental Forces & Moments/Hydrodynamic Forces ==
  "Submarine Velocity (Body Axis) " : Inport
  "AOA, Side Slip" : Inport  Port=2
  Hydrodynamic Forces - Accurate : Subsystem  VariantControl=c==1
  Hydrodynamic Forces - Basic : Subsystem  VariantControl=c==0
  "Force due to Lift, Drag" : Outport  VectorParamsAs1DForOutWhenUnconnected=off

== system AUV_Model/Plant and Environment Model/Environmental Forces & Moments/Hydrostatic Forces ==
  In1 : Inport
  Constant : Constant
  Environment Model : Subsystem  mask{ro=997, V=0.01, M=10, a=0, b=0, c=0}
      mask prompts: ro "Density of Water"; V "Volume of Submarine"; M "Mass of Submarine"; a "X Distance between CG and CB"; b "Y Distance between CG and CB"; c "Z Distance between CG and CB"
      mask DialogControl DescTextVar Prompt: Enter the Submarine related Parameters
      mask DialogControl Container3 Prompt: Distance between CG and Center of Buoyancy
  Hydrostatic Force : Outport  VectorParamsAs1DForOutWhenUnconnected=off
  Hydrostatic Moment : Outport  Port=2  VectorParamsAs1DForOutWhenUnconnected=off
  wires:
  Constant/1 -> Environment Model/1("Fraction submerged ")
  Environment Model/2(Moment due to Weight and Buoyancy) -> Hydrostatic Moment/1
  Environment Model/1(Forces due to Weight and Buoyancy) -> Hydrostatic Force/1
  In1/1 -> Environment Model/2(Orientation Angles)

== system AUV_Model/Plant and Environment Model/Propulsion Forces & Moments/Force and moments due to Thrust ==
  Thrust Inputs : Inport
  "Thrust to Propulsion " : Subsystem
  Propulsion Force : Outport  VectorParamsAs1DForOutWhenUnconnected=off
  Propulsion Moment : Outport  Port=2  VectorParamsAs1DForOutWhenUnconnected=off
  wires:
  "Thrust to Propulsion "/2(Propulsion Moment) -> Propulsion Moment/1
  Thrust Inputs/1 -> "Thrust to Propulsion "/1(Thrust Inputs)
  "Thrust to Propulsion "/1(Propulsion Force) -> Propulsion Force/1

== system AUV_Model/Plant and Environment Model/Propulsion Forces & Moments/Input commands to Thrust ==
  Thrust Control Inputs : Inport
  Demux : Demux  Outputs=3
  Input Commands to PWM : Subsystem
  "PWM Signals to Thrust " : Subsystem
  Thrust values : Outport  VectorParamsAs1DForOutWhenUnconnected=off
  wires:
  Input Commands to PWM/1(Px1) -> "PWM Signals to Thrust "/1(PWM Signal Px1)
  Input Commands to PWM/3(Py1) -> "PWM Signals to Thrust "/3(PWM Signal Py1)
  Demux/1 -> Input Commands to PWM/1(X Thruster)  "X Thrust Input"
  Demux/3 -> Input Commands to PWM/3(Z Thruster)  "Z Thrust Input"
  Input Commands to PWM/4(Py2) -> "PWM Signals to Thrust "/4(PWM Signal Py2)
  Demux/2 -> Input Commands to PWM/2(Y Thruster)  "Y Thrust Input"
  Input Commands to PWM/2(Px2) -> "PWM Signals to Thrust "/2(PWM Signal Px2)
  Input Commands to PWM/5(Pz) -> "PWM Signals to Thrust "/5(PWM Signal Pz)
  "PWM Signals to Thrust "/1(Thrust (N)) -> Thrust values/1
  Thrust Control Inputs/1 -> Demux/1

== system AUV_Model/Sensor data and State Estimation/System With Noise/ Sensor (IMU) ==
  IMU Inputs : Inport
  Bus Creator : BusCreator  Inputs=2
  Bus Selector : BusSelector  OutputSignals=IMU Data
  Demux : Demux  Outputs=5
  Three-axis Inertial Measurement Unit : aerolibnav/Three-axis Inertial Measurement Unit  units=Metric (MKS)  imu=[0 0 0]  i_Ts=0  dtype_a=on  w_a=190  z_a=0.707  a_sf_cc=[1 0 0; 0 1 0; 0 0 1]  a_bias=[0 0 0]  a_sat="[-inf  -inf  -inf  inf inf inf]"  dtype_g=on  w_g=190  z_g=0.707  g_sf_cc=[1 0 0; 0 1 0; 0 0 1]  g_bias=[0 0 0]  g_sens=[0 0 0]  g_sat="[-inf  -inf  -inf  inf inf inf]"  i_rand=on  i_seeds=[23093 23094 23095 23096 23097 23098]  i_pow=[0.00001 0.00001 0.00001 0.00001 0.00001 0.00001]
  IMU Measurements : Outport  VectorParamsAs1DForOutWhenUnconnected=off
  wires:
  Three-axis Inertial Measurement Unit/1 -> Bus Creator/1  "IMU Measured Acceleration"
  Demux/2 -> Three-axis Inertial Measurement Unit/2
  Demux/4 -> Three-axis Inertial Measurement Unit/4
  Demux/5 -> Three-axis Inertial Measurement Unit/5
  Demux/3 -> Three-axis Inertial Measurement Unit/3
  Demux/1 -> Three-axis Inertial Measurement Unit/1
  Three-axis Inertial Measurement Unit/2 -> Bus Creator/2  "IMU Measured Body Rates"
  IMU Inputs/1 -> Bus Selector/1
  Bus Selector/1 -> Demux/1  "<IMU Data>"
  Bus Creator/1 -> IMU Measurements/1

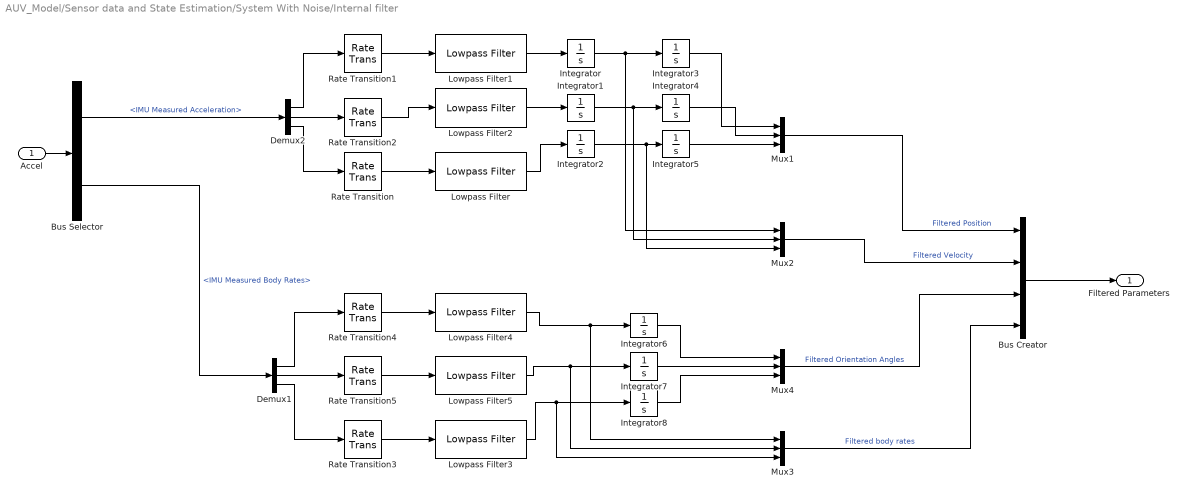
== system AUV_Model/Sensor data and State Estimation/System With Noise/Internal filter ==
  Accel : Inport
  Bus Creator : BusCreator  Inputs=4
  Bus Selector : BusSelector  OutputSignals=IMU Measured Acceleration,IMU Measured Body Rates
  Demux1 : Demux  Outputs=3
  Demux2 : Demux  Outputs=3
  Integrator{,1..8} (9 alike) : Integrator
  Lowpass Filter{,1..5} (6 alike) : dspfdesign/Lowpass Filter  FilterType=FIR  DesignForMinimumOrder=on  FilterOrder=50  PassbandFrequency=1/100  StopbandFrequency=45  PassbandRipple=0.1  StopbandAttenuation=80  InheritSampleRate=off  SampleRate=100  SimulateUsing=Interpreted execution  roundingMode=Floor  coeffsDataTypeStr=fixdt(1,16)
  Mux{1..4} (4 alike) : Mux  Inputs=3
  Rate Transition{,1..5} (6 alike) : RateTransition  OutPortSampleTime=0.01
  Filtered Parameters : Outport  VectorParamsAs1DForOutWhenUnconnected=off
  wires:
  Rate Transition5/1 -> Lowpass Filter5/1
  Rate Transition4/1 -> Lowpass Filter4/1
  Demux1/1 -> Rate Transition4/1
  Lowpass Filter3/1 -> Mux3/3, Integrator8/1
  Demux1/2 -> Rate Transition5/1
  Lowpass Filter5/1 -> Mux3/2, Integrator7/1
  Lowpass Filter4/1 -> Mux3/1, Integrator6/1
  Integrator6/1 -> Mux4/1
  Rate Transition3/1 -> Lowpass Filter3/1
  Integrator8/1 -> Mux4/3
  Demux1/3 -> Rate Transition3/1
  Integrator7/1 -> Mux4/2
  Accel/1 -> Bus Selector/1
  Bus Selector/1 -> Demux2/1  "<IMU Measured Acceleration>"
  Bus Selector/2 -> Demux1/1  "<IMU Measured Body Rates>"
  Mux4/1 -> Bus Creator/3  "Filtered Orientation Angles"
  Mux3/1 -> Bus Creator/4  "Filtered body rates"
  Bus Creator/1 -> Filtered Parameters/1
  Integrator2/1 -> Integrator5/1, Mux2/3
  Integrator/1 -> Mux2/1, Integrator3/1
  Mux2/1 -> Bus Creator/2  "Filtered Velocity"
  Mux1/1 -> Bus Creator/1  "Filtered Position"
  Lowpass Filter/1 -> Integrator2/1
  Demux2/2 -> Rate Transition2/1
  Rate Transition1/1 -> Lowpass Filter1/1
  Integrator4/1 -> Mux1/2
  Demux2/3 -> Rate Transition/1
  Lowpass Filter2/1 -> Integrator1/1
  Lowpass Filter1/1 -> Integrator/1
  Demux2/1 -> Rate Transition1/1
  Integrator5/1 -> Mux1/3
  Integrator1/1 -> Integrator4/1, Mux2/2
  Rate Transition/1 -> Lowpass Filter/1
  Integrator3/1 -> Mux1/1
  Rate Transition2/1 -> Lowpass Filter2/1

== system AUV_Model/Plant and Environment Model/Dynamics solver/Post-Processing/3D Rotate  ==
  "Roll, Pitch, Yaw" : Inport
  Points : Inport  Port=2
  Gain : Gain
  Matrix Multiply : Product  Multiplication=Matrix(*)
  Rotation Angles to Direction Cosine Matrix : sharedtransform/Rotation Angles to Direction Cosine Matrix  rotationOrder=XYZ  aMode=aMode
      settings: SourceProductBaseCode=AE
  Transpose : Math  Operator=transpose  SaturateOnIntegerOverflow=on
  "Transformed " : Outport  VectorParamsAs1DForOutWhenUnconnected=off
  wires:
  Matrix Multiply/1 -> "Transformed "/1
  Rotation Angles to Direction Cosine Matrix/1 -> Transpose/1
  Points/1 -> Matrix Multiply/1
  "Roll, Pitch, Yaw"/1 -> Gain/1
  Transpose/1 -> Matrix Multiply/2
  Gain/1 -> Rotation Angles to Direction Cosine Matrix/1

== system AUV_Model/Plant and Environment Model/Dynamics solver/Post-Processing/3D Rotate Vel ==
  "Roll, Pitch, Yaw" : Inport
  Velocity : Inport  Port=2
  Gain : Gain
  Matrix Multiply : Product  Multiplication=Matrix(*)
  Rotation Angles to Direction Cosine Matrix : sharedtransform/Rotation Angles to Direction Cosine Matrix  rotationOrder=XYZ  aMode=aMode
      settings: SourceProductBaseCode=AE
  Transpose : Math  Operator=transpose  SaturateOnIntegerOverflow=on
  "Transformed_velocity " : Outport  VectorParamsAs1DForOutWhenUnconnected=off
  wires:
  Matrix Multiply/1 -> "Transformed_velocity "/1
  Rotation Angles to Direction Cosine Matrix/1 -> Transpose/1
  Velocity/1 -> Matrix Multiply/2
  "Roll, Pitch, Yaw"/1 -> Gain/1
  Transpose/1 -> Matrix Multiply/1
  Gain/1 -> Rotation Angles to Direction Cosine Matrix/1

== system AUV_Model/Plant and Environment Model/Environmental Forces & Moments/Hydrodynamic Forces/Hydrodynamic Forces - Accurate ==
  note: Source of Equations:
      | Submarine Dynamic Modeling, by
      | Dr Peter Ridley Julien Fontan and Dr Peter Corke
      |
      | Part: Hydrodynamic forces and moments
  "Submarine Velocity (Body Axis) " : Inport
  "AOA, Side Slip" : Inport  Port=2
  Force Exerted due to Drag (Body Axis) : Subsystem
  Force Exerted due to Lift (Body Axis) : Subsystem
  Sum : Sum
  "Force due to Lift, Drag" : Outport  VectorParamsAs1DForOutWhenUnconnected=off
  wires:
  Force Exerted due to Drag (Body Axis)/1(Drag Forces in Body Axis) -> Sum/1
  Force Exerted due to Lift (Body Axis)/1(Lift Forces in Body Axis) -> Sum/2
  "AOA, Side Slip"/1 -> Force Exerted due to Drag (Body Axis)/2(AOA and Side Slip), Force Exerted due to Lift (Body Axis)/2(AOA and Side Slip)
  "Submarine Velocity (Body Axis) "/1 -> Force Exerted due to Lift (Body Axis)/1(Marine Velocities in Body Axis), Force Exerted due to Drag (Body Axis)/1(Marine Velocities in Body Axis)
  Sum/1 -> "Force due to Lift, Drag"/1

== system AUV_Model/Plant and Environment Model/Environmental Forces & Moments/Hydrodynamic Forces/Hydrodynamic Forces - Basic ==
  "Submarine Velocity (Body Axis) " : Inport
  "AOA, Side Slip" : Inport  Port=2
  Force Exerted due to Drag (Body Axis) : Subsystem
  Force Exerted due to Lift (Body Axis) : Subsystem
  Sum : Sum
  "Force due to Lift, Drag" : Outport  VectorParamsAs1DForOutWhenUnconnected=off
  wires:
  Force Exerted due to Drag (Body Axis)/1(Drag Forces in Body Axis) -> Sum/1
  Force Exerted due to Lift (Body Axis)/1(Lift Forces in Body Axis) -> Sum/2
  "AOA, Side Slip"/1 -> Force Exerted due to Drag (Body Axis)/2(AOA and Side Slip), Force Exerted due to Lift (Body Axis)/2(AOA and Side Slip)
  "Submarine Velocity (Body Axis) "/1 -> Force Exerted due to Lift (Body Axis)/1(Marine Velocities in Body Axis), Force Exerted due to Drag (Body Axis)/1(Marine Velocities in Body Axis)
  Sum/1 -> "Force due to Lift, Drag"/1

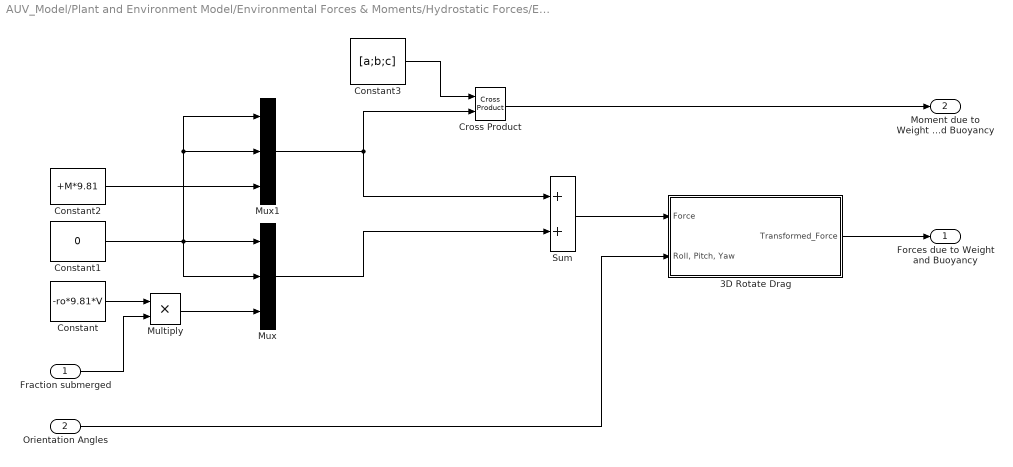
== system AUV_Model/Plant and Environment Model/Environmental Forces & Moments/Hydrostatic Forces/Environment Model ==
  "Fraction submerged " : Inport
  Orientation Angles : Inport  Port=2
  3D Rotate Drag : Subsystem
  Constant : Constant  Value=-ro*9.81*V
  Constant1 : Constant  Value=0
  Constant2 : Constant  Value=+M*9.81
  Constant3 : Constant  Value=[a;b;c]
  Cross Product : vrlib/Utilities/Cross Product
      settings: SourceProductBaseCode=VR
  Multiply : Product
  Mux : Mux  Inputs=3
  Mux1 : Mux  Inputs=3
  Sum : Sum
  Forces due to Weight and Buoyancy : Outport  VectorParamsAs1DForOutWhenUnconnected=off
  Moment due to Weight and Buoyancy : Outport  Port=2  VectorParamsAs1DForOutWhenUnconnected=off
  wires:
  Cross Product/1 -> Moment due to Weight and Buoyancy/1
  Constant3/1 -> Cross Product/1
  "Fraction submerged "/1 -> Multiply/2
  Mux/1 -> Sum/2
  Multiply/1 -> Mux/3
  Mux1/1 -> Sum/1, Cross Product/2
  Constant/1 -> Multiply/1
  Constant1/1 -> Mux/1, Mux/2, Mux1/2, Mux1/1
  Constant2/1 -> Mux1/3
  Sum/1 -> 3D Rotate Drag/1(Force)
  Orientation Angles/1 -> 3D Rotate Drag/2("Roll, Pitch, Yaw")
  3D Rotate Drag/1("Transformed_Force ") -> Forces due to Weight and Buoyancy/1

== system AUV_Model/Plant and Environment Model/Propulsion Forces & Moments/Force and moments due to Thrust/Thrust to Propulsion  ==
  Thrust Inputs : Inport
  Demux : Demux  Outputs=5
  Moment computation : Subsystem
  Sum : Sum  Inputs=+++++
  Thrust Transformation : Subsystem
  Propulsion Force : Outport  VectorParamsAs1DForOutWhenUnconnected=off
  Propulsion Moment : Outport  Port=2  VectorParamsAs1DForOutWhenUnconnected=off
  wires:
  Demux/5 -> Moment computation/5(Pz)
  Demux/4 -> Moment computation/4(Py2)
  Demux/3 -> Moment computation/3(Py1)
  Demux/2 -> Moment computation/2(Px2)
  Demux/1 -> Moment computation/1(Px1)
  Thrust Transformation/3(Thrust Py1) -> Sum/3
  Moment computation/1(Moment) -> Propulsion Moment/1
  Thrust Transformation/4(Thrust Py2) -> Sum/4
  Thrust Transformation/5(Thrust Pz) -> Sum/5
  Sum/1 -> Propulsion Force/1
  Thrust Inputs/1 -> Thrust Transformation/1(Thrust Inputs), Demux/1
  Thrust Transformation/1(Thrust Px1) -> Sum/1
  Thrust Transformation/2(Thrust Px2) -> Sum/2

== system AUV_Model/Plant and Environment Model/Propulsion Forces & Moments/Input commands to Thrust/Input Commands to PWM ==
  X Thruster : Inport
  Y Thruster : Inport  Port=2
  Z Thruster : Inport  Port=3
  1-D Lookup Table : Lookup_n-D  NumberOfTableDimensions=1  BreakpointsForDimension1=[-1:0.01:1]  Table=1500 + 400 * ([-1:0.01:1])  InternalRulePriority=Speed  RndMeth=Simplest  InputSameDT=on
  1-D Lookup Table1 : Lookup_n-D  NumberOfTableDimensions=1  BreakpointsForDimension1=[-1:0.01:1]  Table=1500 + 400 * ([-1:0.01:1])  InternalRulePriority=Speed  RndMeth=Simplest  InputSameDT=on
  1-D Lookup Table2 : Lookup_n-D  NumberOfTableDimensions=1  BreakpointsForDimension1=[-1:0.01:1]  Table=1500 + 400 * ([-1:0.01:1])  InternalRulePriority=Speed  RndMeth=Simplest  InputSameDT=on
  Px1 : Outport  VectorParamsAs1DForOutWhenUnconnected=off
  Px2 : Outport  Port=2  VectorParamsAs1DForOutWhenUnconnected=off
  Py1 : Outport  Port=3  VectorParamsAs1DForOutWhenUnconnected=off
  Py2 : Outport  Port=4  VectorParamsAs1DForOutWhenUnconnected=off
  Pz : Outport  Port=5  VectorParamsAs1DForOutWhenUnconnected=off
  wires:
  1-D Lookup Table2/1 -> Pz/1
  Y Thruster/1 -> 1-D Lookup Table1/1
  1-D Lookup Table1/1 -> Py1/1, Py2/1
  1-D Lookup Table/1 -> Px1/1, Px2/1
  Z Thruster/1 -> 1-D Lookup Table2/1
  X Thruster/1 -> 1-D Lookup Table/1

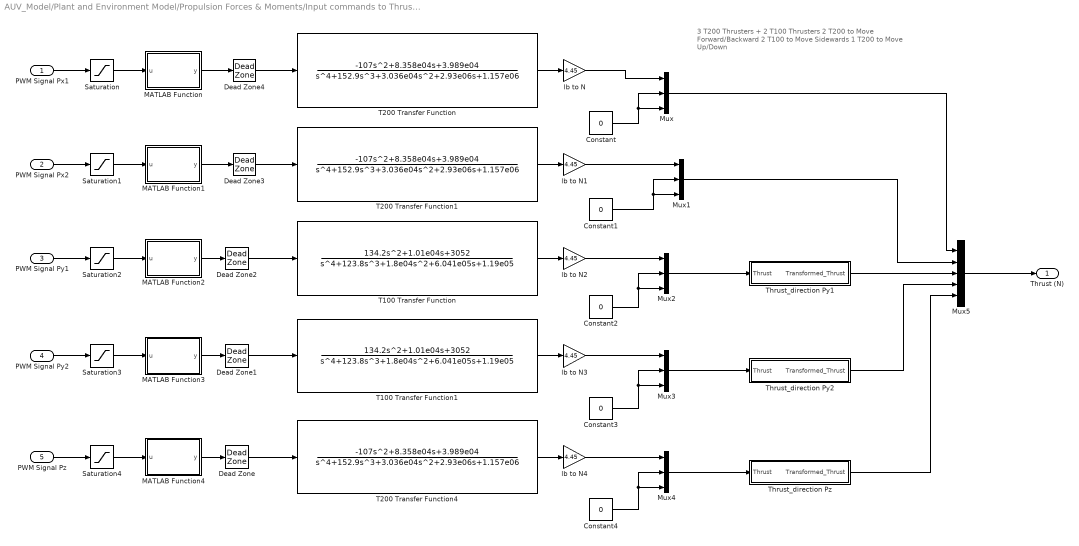
== system AUV_Model/Plant and Environment Model/Propulsion Forces & Moments/Input commands to Thrust/PWM Signals to Thrust  ==
  note: 3 T200 Thrusters + 2 T100 Thrusters
      |
      | 2 T200 to Move Forward/Backward
      | 2 T100 to Move Sidewards
      | 1 T200 to Move Up/Down
  PWM Signal Px1 : Inport
  PWM Signal Px2 : Inport  Port=2
  PWM Signal Py1 : Inport  Port=3
  PWM Signal Py2 : Inport  Port=4
  PWM Signal Pz : Inport  Port=5
  Constant{,1..4} (5 alike) : Constant  Value=0
  Dead Zone{,2..4} (4 alike) : DeadZone  LowerValue=-10  UpperValue=+10  SaturateOnIntegerOverflow=on
  Dead Zone1 : DeadZone  LowerValue=-10  UpperValue=10  SaturateOnIntegerOverflow=on
  MATLAB Function : MATLAB Function  TreatAsAtomicUnit=on
  MATLAB Function1 : MATLAB Function  TreatAsAtomicUnit=on
  MATLAB Function2 : MATLAB Function  TreatAsAtomicUnit=on
  MATLAB Function3 : MATLAB Function  TreatAsAtomicUnit=on
  MATLAB Function4 : MATLAB Function  TreatAsAtomicUnit=on
  Mux{,1..4} (5 alike) : Mux  Inputs=3
  Mux5 : Mux  Inputs=5
  Saturation{,1..4} (5 alike) : Saturate  UpperLimit=1900  LowerLimit=1100
  T100 Transfer Function : TransferFcn  Numerator="[134.2 1.01e04  3052]"  Denominator=[1 123.8 1.8e04 6.041e05 1.19e05]
  T100 Transfer Function1 : TransferFcn  Numerator="[134.2 1.01e04  3052]"  Denominator=[1 123.8 1.8e04 6.041e05 1.19e05]
  T200 Transfer Function : TransferFcn  Numerator="[-107  8.358e04  3.989e04]"  Denominator="[1 152.9  3.036e04  2.93e06  1.157e06]"
  T200 Transfer Function1 : TransferFcn  Numerator="[-107  8.358e04  3.989e04]"  Denominator="[1 152.9  3.036e04  2.93e06  1.157e06]"
  T200 Transfer Function4 : TransferFcn  Numerator="[-107  8.358e04  3.989e04]"  Denominator="[1 152.9  3.036e04  2.93e06  1.157e06]"
  Thrust_direction Py1 : Subsystem
  Thrust_direction Py2 : Subsystem
  Thrust_direction Pz : Subsystem
  lb to N{,1..4} (5 alike) : Gain  Gain=4.45
  Thrust (N) : Outport  VectorParamsAs1DForOutWhenUnconnected=off
  wires:
  Dead Zone4/1 -> T200 Transfer Function/1
  Dead Zone3/1 -> T200 Transfer Function1/1
  Dead Zone2/1 -> T100 Transfer Function/1
  Dead Zone1/1 -> T100 Transfer Function1/1
  Dead Zone/1 -> T200 Transfer Function4/1
  MATLAB Function4/1(y) -> Dead Zone/1
  MATLAB Function3/1(y) -> Dead Zone1/1
  MATLAB Function2/1(y) -> Dead Zone2/1
  MATLAB Function1/1(y) -> Dead Zone3/1
  Saturation3/1 -> MATLAB Function3/1(u)
  PWM Signal Py2/1 -> Saturation3/1
  Saturation4/1 -> MATLAB Function4/1(u)
  Saturation2/1 -> MATLAB Function2/1(u)
  Saturation1/1 -> MATLAB Function1/1(u)
  Saturation/1 -> MATLAB Function/1(u)
  MATLAB Function/1(y) -> Dead Zone4/1
  T100 Transfer Function1/1 -> lb to N3/1
  lb to N2/1 -> Mux2/1
  Mux4/1 -> Thrust_direction Pz/1(Thrust)
  Mux5/1 -> Thrust (N)/1
  Thrust_direction Pz/1("Transformed_Thrust ") -> Mux5/5
  lb to N/1 -> Mux/1
  Constant1/1 -> Mux1/2, Mux1/3
  T200 Transfer Function1/1 -> lb to N1/1
  Mux3/1 -> Thrust_direction Py2/1(Thrust)
  PWM Signal Pz/1 -> Saturation4/1
  PWM Signal Px1/1 -> Saturation/1
  Constant/1 -> Mux/2, Mux/3
  Thrust_direction Py2/1("Transformed_Thrust ") -> Mux5/4
  Thrust_direction Py1/1("Transformed_Thrust ") -> Mux5/3
  PWM Signal Py1/1 -> Saturation2/1
  Mux1/1 -> Mux5/2
  lb to N1/1 -> Mux1/1
  lb to N4/1 -> Mux4/1
  Constant4/1 -> Mux4/2, Mux4/3
  T200 Transfer Function4/1 -> lb to N4/1
  Mux/1 -> Mux5/1
  T200 Transfer Function/1 -> lb to N/1
  Constant2/1 -> Mux2/2, Mux2/3
  Mux2/1 -> Thrust_direction Py1/1(Thrust)
  PWM Signal Px2/1 -> Saturation1/1
  Constant3/1 -> Mux3/2, Mux3/3
  lb to N3/1 -> Mux3/1
  T100 Transfer Function/1 -> lb to N2/1
